simulink model "test_fas_fbs_fcs"  (R2022b)
settings: Solver=VariableStepAuto  StartTime=0.0  StopTime=1  MaxStep=0.001  RelTol=1e-3
settings Model: Creator=jack  LastModifiedBy=jack

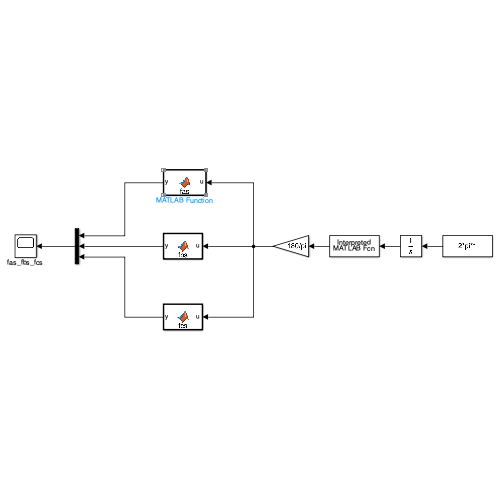
[thumbnail: Simulink's stored preview of the top-level diagram]
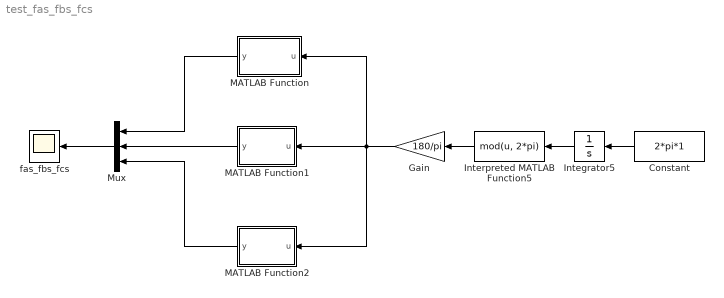
== system test_fas_fbs_fcs ==
  Constant : Constant  Value=2*pi*1
  Gain : Gain  Gain=180/pi
  Integrator5 : Integrator
  Interpreted MATLAB Function5 : MATLABFcn  MATLABFcn=mod(u, 2*pi)
  MATLAB Function : MATLAB Function  TreatAsAtomicUnit=on
  MATLAB Function1 : MATLAB Function  TreatAsAtomicUnit=on
  MATLAB Function2 : MATLAB Function  TreatAsAtomicUnit=on
  Mux : Mux  Inputs=3
  fas_fbs_fcs : Scope
  wires:
  Integrator5/1 -> Interpreted MATLAB Function5/1
  Constant/1 -> Integrator5/1
  Interpreted MATLAB Function5/1 -> Gain/1
  MATLAB Function/1(y) -> Mux/1
  Mux/1 -> fas_fbs_fcs/1
  Gain/1 -> MATLAB Function2/1(u), MATLAB Function/1(u), MATLAB Function1/1(u)
  MATLAB Function1/1(y) -> Mux/2
  MATLAB Function2/1(y) -> Mux/3

== matlab function test_fas_fbs_fcs/MATLAB Function ==
  data: u input; y output
function y = fas(u)
    if ((u>=0) && (u<30))
        y = u/30;
    elseif ((u>=30) && (u<150))
        y = 1;
    elseif ((u>=150) && (u<210))
        y = -u/30 + 6;
    elseif ((u>=210) && (u<330))
        y = -1;
    elseif ((u>=330) && (u<=360))
        y = u/30 - 12;
    else
        y = 0;
    end
end

== matlab function test_fas_fbs_fcs/MATLAB Function2 ==
  data: u input; y output
function y = fcs(u)
    if ((u>=0) && (u<30))
        y = 1;
    elseif ((u>=30) && (u<90))
        y = -u/30 + 2;
    elseif ((u>=90) && (u<210))
        y = -1;
    elseif ((u>=210) && (u<270))
        y = u/30 - 8;
    elseif ((u>=270) && (u<=360))
        y = 1;
    else 
        y = 0;
    end
end

== matlab function test_fas_fbs_fcs/MATLAB Function1 ==
  data: u input; y output
function y = fbs(u)
    if ((u>=0) && (u<90))
        y = -1;
    elseif ((u>=90) && (u<150))
        y = u/30 - 4;
    elseif ((u>=150) && (u<270))
        y = 1;
    elseif ((u>=270) && (u<330))
        y = -u/30 + 10;
    elseif ((u>=330) && (u<=360))
        y = -1;
    else
        y = 0;
    end
end
